simulink model "uuvSim"  (R2017a)
settings: Solver=ode4  StartTime=0.0  StopTime=10.0  FixedStep=mdl.tStep  RelTol=1e-3
undefined symbols (not defined in the file): ics, rov, tau, v_c
settings Model: Creator=e_anderlini  LastModifiedBy=e_anderlini

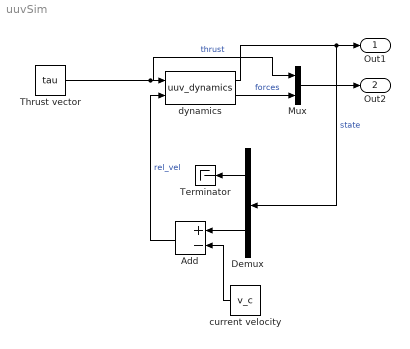
== system uuvSim ==
  Add : Sum  Inputs=+-
  Demux : Demux  Outputs=[6,6]
  Mux : Mux  Inputs=[6,12]
  Terminator : Terminator
  Thrust vector : Constant  Value=tau
  current velocity : Constant  Value=v_c
  dynamics : S-Function  FunctionName=uuv_dynamics  Parameters=rov.weight,rov.buoyancy,rov.G,rov.B,ics,rov.inv_mass',rov.D_L',rov.D_q'  SFunctionDeploymentMode=off  EnableBusSupport=off
  Out1 : Outport
  Out2 : Outport  Port=2
  wires:
  dynamics/1 -> Demux/1, Out1/1  "state"
  Demux/1 -> Terminator/1
  Add/1 -> dynamics/2  "rel_vel"
  current velocity/1 -> Add/2
  Demux/2 -> Add/1
  Mux/1 -> Out2/1
  dynamics/2 -> Mux/2  "forces"
  Thrust vector/1 -> Mux/1, dynamics/1  "thrust"
